simulink model "Sikmy_vrh_2"  (Simulink 8.6)
settings: Solver=ode45  StartTime=0.0  StopTime=td  MaxStep=0.01  RelTol=1e-3
values from neighbouring files (symbols this model uses):
  alfa_rad = alfa_deg*2*pi/360    (= 1.0471975512)    [Sikmy_vrh_par.m]
  g = 9.81    [Sikmy_vrh_par.m]
  v0 = 50    [Sikmy_vrh_par.m]
libraries: tos_lib x1
settings Model: Creator=Igor Belai  LastModifiedBy=Erich
settings DataIOCC: LimitDataPoints=off
settings OptimizationCC: InitFltsAndDblsToZero=on
settings DebuggingCC: FcnCallInpInsideContextMsg=UseLocalSettings

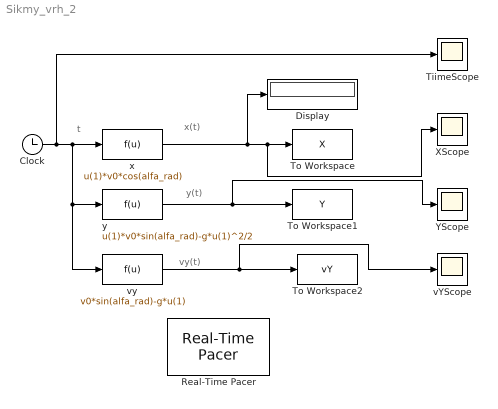
== system Sikmy_vrh_2 ==
  note: t
  note: y(t)
  note: x(t)
  note: vy(t)
  Clock : Clock
  Display : Display
  Real-Time Pacer : tos_lib/Real-Time Pacer  simTimePerRealTime=1
  TiimeScope : Scope
  To Workspace : ToWorkspace  VariableName=X
  To Workspace1 : ToWorkspace  VariableName=Y  SampleTime=-1
  To Workspace2 : ToWorkspace  VariableName=vY  SampleTime=-1
  "XScope " : Scope
  "YScope " : Scope
  vYScope : Scope
  vy : Fcn  Expr=v0*sin(alfa_rad)-g*u(1)
  x : Fcn  Expr=u(1)*v0*cos(alfa_rad)
  y : Fcn  Expr=u(1)*v0*sin(alfa_rad)-g*u(1)^2/2
  wires:
  Clock/1 -> TiimeScope/1, x/1, y/1, vy/1
  x/1 -> Display/1, "XScope "/1, To Workspace/1
  y/1 -> To Workspace1/1, "YScope "/1
  vy/1 -> vYScope/1, To Workspace2/1
